simulink library "templibrary"  (Simulink 4.00)
undefined symbols (not defined in the file or in its folder): sfunxyauto
settings Model: LastModifiedBy=galoe

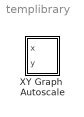
== system templibrary ==
  XY Graph  Autoscale : Subsystem  LoadFcn=sfunxyauto([],[],[],'LoadBlock')  StartFcn=sfunxyauto([],[],[],'Start')  StopFcn=sfunxyauto([],[],[],'Stop')  TreatAsAtomicUnit=on  SimViewingDevice=on  mask(XY scope.){xmin=-1, xmax=1, ymin=-1, ymax=1, st=-1}
      mask prompts: xmin "x-min:"; xmax "x-max:"; ymin "y-min:"; ymax "y-max:"; st "Sample time:"
      mask help: XY scope using MATLAB graph window. First input is used as time base. Enter plotting ranges.
      settings: CopyFcn=sfunxyauto([],[],[],'CopyBlock')  DeleteFcn=sfunxyauto([],[],[],'DeleteBlock')  NameChangeFcn=sfunxyauto([],[],[],'NameChange')  RTWFcnNameOpts=Auto  RTWFileNameOpts=Auto
      mask Help: This block can be used to explore limit cycles. Look at the m-file sfunxy.m to see how it works.
      mask Display: plot([.05 .95 .95 .05 .05],[.45 .45 .95 .95 .45], 0.5+cos(0:0.1:2*pi)*0.3,0.7+sin(0:0.1:2*pi)*0.2)

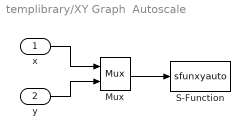
== system templibrary/XY Graph  Autoscale ==
  x : Inport  Port=1  LatchInput=off
  y : Inport  Port=2  LatchInput=off
  Mux : Mux  Inputs=2
      settings: DisplayOption=none
  S-Function : S-Function  FunctionName=sfunxyauto  Parameters=[xmin xmax ymin ymax], st  PortCounts=[]  SFunctionModules=''
  wires:
  Mux/1 -> S-Function/1
  x/1 -> Mux/1
  y/1 -> Mux/2
